simulink model "draw_aircraft_sim"  (R2023b)
settings: Solver=FixedStepDiscrete  StartTime=0.0  StopTime=1E4  FixedStep=0.2  RelTol=1e-3
undefined symbols (not defined in the file or in its folder): draw_aircraft
libraries: simulink x8
settings Model: Creator=pf  LastModifiedBy=piotr

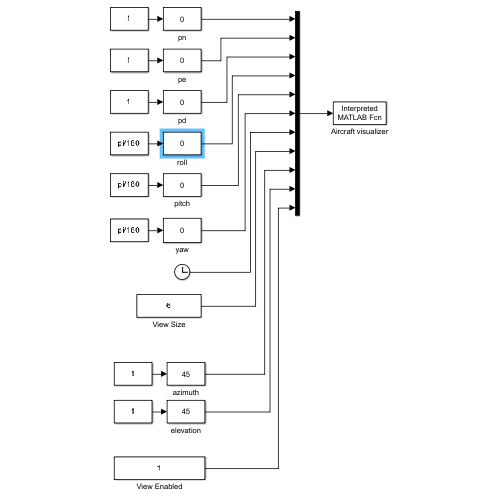
[thumbnail: Simulink's stored preview of the top-level diagram]
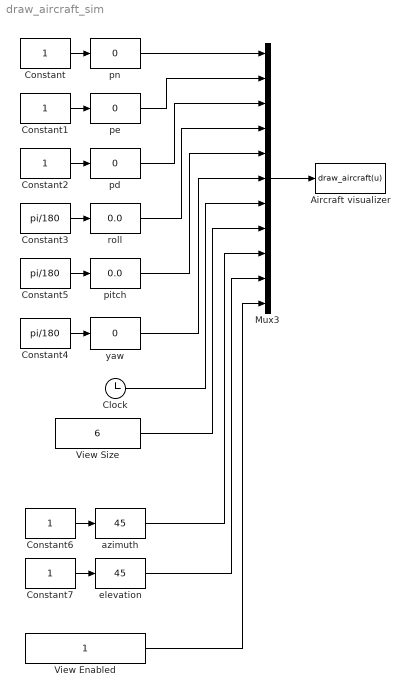
== system draw_aircraft_sim ==
  Aircraft visualizer : MATLABFcn  MATLABFcn=draw_aircraft(u)  OutputDimensions=0
  Clock : Clock
  Constant{,1..2,6..7} (5 alike) : Constant
  Constant3 : Constant  Value=pi/180
  Constant4 : Constant  Value=pi/180
  Constant5 : Constant  Value=pi/180
  Mux3 : Mux  Inputs=11
  View Enabled : Constant
  View Size : Constant  Value=6
  azimuth : simulink/Math Operations/Slider Gain  gain=45  low=-180  high=180
  elevation : simulink/Math Operations/Slider Gain  gain=45  low=-180  high=180
  pd : simulink/Math Operations/Slider Gain  gain=0  low=-12  high=12
  pe : simulink/Math Operations/Slider Gain  gain=0  low=-12  high=12
  pitch : simulink/Math Operations/Slider Gain  gain=0.0  low=-90  high=90
  pn : simulink/Math Operations/Slider Gain  gain=0  low=-12  high=12
  roll : simulink/Math Operations/Slider Gain  gain=0.0  low=-180  high=180
  yaw : simulink/Math Operations/Slider Gain  gain=0  low=-180  high=180
  wires:
  Constant/1 -> pn/1
  Constant1/1 -> pe/1
  Constant2/1 -> pd/1
  pn/1 -> Mux3/1
  pe/1 -> Mux3/2
  pd/1 -> Mux3/3
  Constant3/1 -> roll/1
  roll/1 -> Mux3/4
  Constant4/1 -> yaw/1
  Constant5/1 -> pitch/1
  pitch/1 -> Mux3/5
  yaw/1 -> Mux3/6
  Constant7/1 -> elevation/1
  Constant6/1 -> azimuth/1
  Clock/1 -> Mux3/7
  Mux3/1 -> Aircraft visualizer/1
  View Size/1 -> Mux3/8
  azimuth/1 -> Mux3/9
  elevation/1 -> Mux3/10
  View Enabled/1 -> Mux3/11
